simulink model "fuzzytfg3"  (R2020b)
settings: Solver=ode5  StartTime=0.0  StopTime=inf  RelTol=1e-3
undefined symbols (not defined in the file): National_Instruments, PCI
libraries: sldrtlib x2, fuzblock x1
settings Model: SimulationMode=external  Creator=Usuario_UMA  LastModifiedBy=alumnoic03
settings RTWCC: Description=Simulink Desktop Real-Time  SystemTargetFile=sldrt.tlc  TemplateMakefile=sldrt.tmf  RTWCompilerOptimization=on
settings CodeAppCC: MaxIdLength=95
settings SimulinkDesktopRealTimeCC: TargetPreCompLibLocation=C:\Program Files\MATLAB\R2020\toolbox\sldrt\lib\win64

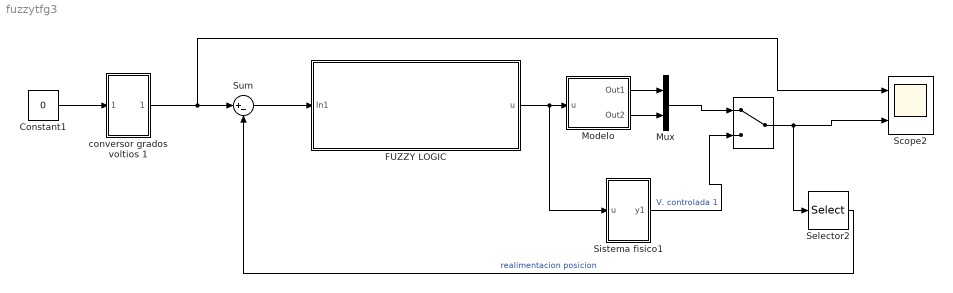
== system fuzzytfg3 ==
  " " : ManualSwitch
  Constant1 : Constant  Value=0
  FUZZY LOGIC : Subsystem
  "Modelo " : Subsystem
  Mux : Mux  Inputs=2
  Scope2 : Scope  NumInputPorts=2
  Selector2 : Selector  InputPortWidth=2  IndexOptions=Index vector (dialog)  Indices=[1]  OutputSizes=1
  Sistema fisico1 : Subsystem
  Sum : Sum  Inputs=|+-
  conversor grados voltios 1 : Subsystem  mask{a=4.95, b=0}
  wires:
  Sistema fisico1/1(y1) -> " "/2  "V. controlada 1"
  Constant1/1 -> conversor grados voltios 1/1(In1)
  conversor grados voltios 1/1(Out1) -> Sum/1, Scope2/1
  FUZZY LOGIC/1(u) -> Sistema fisico1/1(u), "Modelo "/1(u)
  Selector2/1 -> Sum/2  "realimentacion posicion"
  Sum/1 -> FUZZY LOGIC/1(In1)
  "Modelo "/2(Out2) -> Mux/2
  "Modelo "/1(Out1) -> Mux/1
  " "/1 -> Selector2/1, Scope2/2
  Mux/1 -> " "/1

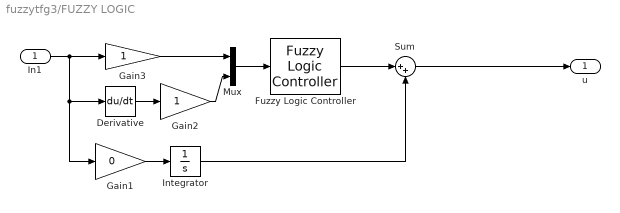
== system fuzzytfg3/FUZZY LOGIC ==
  In1 : Inport
  Derivative : Derivative
  Fuzzy Logic Controller : fuzblock/Fuzzy Logic  Controller  FIS='FUZZY4.fis'  OutputSampleNumber=101  DataType=double  FuzzifiedInputs=off  RuleFiringStrengths=off  RuleOutputs=off  AggregatedOutputs=off  SimulateUsing=Interpreted execution  OutOfRangeInputValueMessage=warning  NoRuleFiredMessage=warning  EmptyOutputFuzzySetMessage=warning
  Gain1 : Gain  Gain=0
  Gain2 : Gain
  Gain3 : Gain
  Integrator : Integrator
  Mux : Mux  Inputs=2
  Sum : Sum  Inputs=|++
  u : Outport
  wires:
  In1/1 -> Gain3/1, Gain1/1, Derivative/1
  Mux/1 -> Fuzzy Logic Controller/1
  Gain3/1 -> Mux/1
  Derivative/1 -> Gain2/1
  Gain2/1 -> Mux/2
  Gain1/1 -> Integrator/1
  Fuzzy Logic Controller/1 -> Sum/1
  Integrator/1 -> Sum/2
  Sum/1 -> u/1

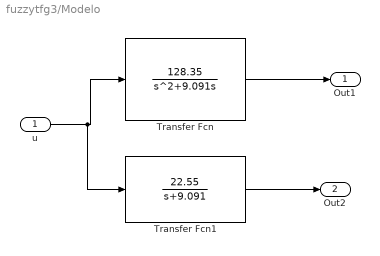
== system fuzzytfg3/Modelo  ==
  u : Inport
  Transfer Fcn : TransferFcn  Numerator=[128.35]  Denominator=[1 9.091 0]
  Transfer Fcn1 : TransferFcn  Numerator=[22.55]  Denominator=[1 9.091]
  Out1 : Outport
  Out2 : Outport  Port=2
  wires:
  u/1 -> Transfer Fcn1/1, Transfer Fcn/1
  Transfer Fcn/1 -> Out1/1
  Transfer Fcn1/1 -> Out2/1

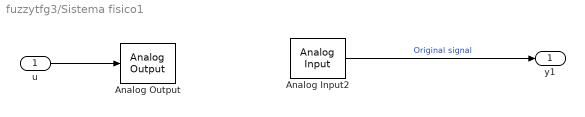
== system fuzzytfg3/Sistema fisico1 ==
  u : Inport
  Analog Input2 : sldrtlib/Analog Input  SampleTime=0.001  MaxMissedTicks=10  ShowMissedTicks=off  YieldWhenWaiting=off  DrvName=National_Instruments/PCI-6014  DrvAddress=4294967295  DrvOptions=[2 0 0 0 0 0]  Channels=[1,2]  RangeMode=1  VoltRange=1  DataType=1
      settings: AttributesFormatString=National Instruments\nPCI-6014 [auto]
  Analog Output : sldrtlib/Analog Output  SampleTime=0.001  MaxMissedTicks=10  ShowMissedTicks=off  YieldWhenWaiting=off  DrvName=National_Instruments/PCI-6014  DrvAddress=4294967295  DrvOptions=[2 0 0 0 0 0]  Channels=1  RangeMode=1  VoltRange=1  InitialValue=[]  FinalValue=[]
      settings: AttributesFormatString=National Instruments\nPCI-6014 [auto]
  y1 : Outport
  wires:
  u/1 -> Analog Output/1
  Analog Input2/1 -> y1/1  "Original signal"

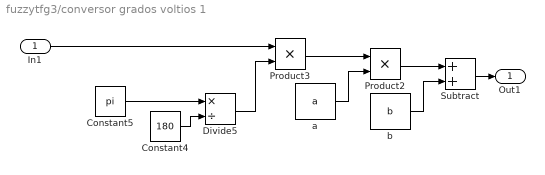
== system fuzzytfg3/conversor grados voltios 1 ==
  In1 : Inport
  Constant4 : Constant  Value=180
  Constant5 : Constant  Value=pi
  Divide5 : Product  Inputs=*/
  Product2 : Product
  Product3 : Product
  Subtract : Sum
  a : Constant  Value=a
  b : Constant  Value=b
  Out1 : Outport
  wires:
  b/1 -> Subtract/2
  Product3/1 -> Product2/1
  Constant4/1 -> Divide5/2
  In1/1 -> Product3/1
  Product2/1 -> Subtract/1
  a/1 -> Product2/2
  Constant5/1 -> Divide5/1
  Divide5/1 -> Product3/2
  Subtract/1 -> Out1/1
